simulink model "VTOL_DigitalPID"  (R2016b)
settings: Solver=ode45  StartTime=0.0  StopTime=500  RelTol=1e-3  EnableMultiTasking=on
InitFcn:
  | param
undefined symbols (not defined in the file or in its folder): drawVTOLsys, P, VTOL_ctrl_state_int
settings Model: Creator=beard  LastModifiedBy=Jacob
settings DataIOCC: LimitDataPoints=on  SaveFormat=Array  SignalLoggingSaveFormat=ModelDataLogs
settings OptimizationCC: ExpressionDepthLimit=2147483647  InitFltsAndDblsToZero=on  LifeSpan=inf
settings DebuggingCC: UnderspecifiedInitializationDetection=Classic  MergeDetectMultiDrivingBlocksExec=none  SolverPrmCheckMsg=warning  FcnCallInpInsideContextMsg=warning  StateNameClashWarn=warning  SFUnexpectedBacktrackingDiag=warning  SFNoUnconditionalDefaultTransitionDiag=warning  SFExecutionAtInitializationDiag=none
settings HardwareCC: ProdBitPerPointer=32  ProdBitPerSizeT=32  ProdBitPerPtrDiffT=32  ProdLargestAtomicFloat=None  ProdIntDivRoundTo=Undefined  ProdEndianess=Unspecified  ProdWordSize=32  ProdHWDeviceType=32-bit Generic
settings ModelReferenceCC: PropagateSignalLabelsOutOfModel=off
settings GRTTargetCC: TargetLangStandard=C89/C90 (ANSI)  GeneratePreprocessorConditionals=Disable all  CombineOutputUpdateFcns=off  GRTInterface=on
settings ConfigComp: CovMetricSettings=dw  CovHtmlReporting=on  CovSaveCumulativeToWorkspaceVar=on  CovSaveSingleToWorkspaceVar=on  CovExternalEMLEnable=off

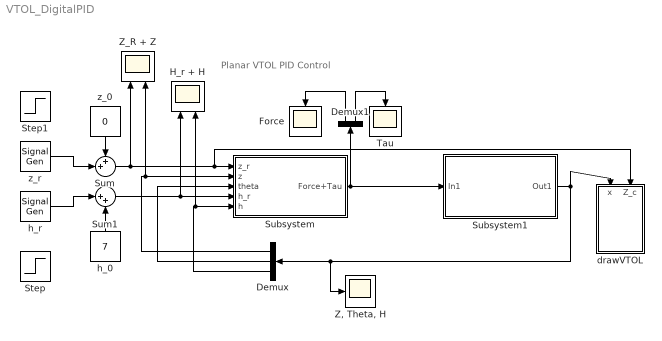
== system VTOL_DigitalPID ==
  note: Planar VTOL PID Control
  Demux : Demux  Outputs=3
  Demux1 : Demux  Outputs=2
  Force : Scope
  H_r + H : Scope  NumInputPorts=2
  Step : Step  After=3  SampleTime=0
  Step1 : Step  After=2  SampleTime=0
  Subsystem : Subsystem
  Subsystem1 : Subsystem
  Sum : Sum  Inputs=++|
  Sum1 : Sum  Inputs=|++
  Tau : Scope
  "Z, Theta, H" : Scope
  Z_R + Z : Scope  NumInputPorts=2
  drawVTOL : Subsystem
  h_0 : Constant  Value=7
  h_r : SignalGenerator  WaveForm=square  Amplitude=5  Frequency=.01
  z_0 : Constant  Value=0
  z_r : SignalGenerator  WaveForm=square  Amplitude=5  Frequency=0.015
  wires:
  z_0/1 -> Sum/1
  h_0/1 -> Sum1/2
  Sum/1 -> drawVTOL/2(Z_c), Subsystem/1(z_r), Z_R + Z/1
  Demux/1 -> Subsystem/2(z), Z_R + Z/2
  Demux/2 -> Subsystem/3(theta)
  Demux/3 -> Subsystem/5(h), H_r + H/2
  Sum1/1 -> Subsystem/4(h_r), H_r + H/1
  h_r/1 -> Sum1/1
  z_r/1 -> Sum/2
  Demux1/2 -> Tau/1
  Demux1/1 -> Force/1
  Subsystem/1(Force+Tau) -> Subsystem1/1(In1), Demux1/1
  Subsystem1/1(Out1) -> "Z, Theta, H"/1, Demux/1, drawVTOL/1(x)

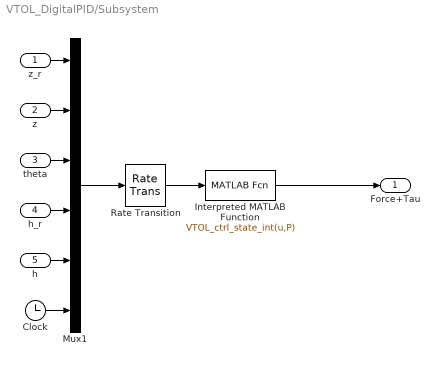
== system VTOL_DigitalPID/Subsystem ==
  z_r : Inport
  z : Inport  Port=2
  theta : Inport  Port=3
  h_r : Inport  Port=4
  h : Inport  Port=5
  Clock : Clock
  Interpreted MATLAB Function : MATLABFcn  MATLABFcn=VTOL_ctrl_state_int(u,P)  OutputDimensions=2  Output1D=off
  Mux1 : Mux  Inputs=6
  Rate Transition : RateTransition  OutPortSampleTime=P.Ts
  Force+Tau : Outport
  wires:
  Rate Transition/1 -> Interpreted MATLAB Function/1
  Mux1/1 -> Rate Transition/1
  z_r/1 -> Mux1/1
  h_r/1 -> Mux1/4
  theta/1 -> Mux1/3
  z/1 -> Mux1/2
  h/1 -> Mux1/5
  Clock/1 -> Mux1/6
  Interpreted MATLAB Function/1 -> Force+Tau/1

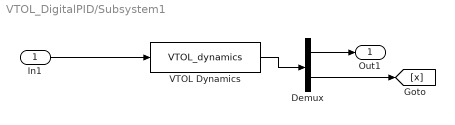
== system VTOL_DigitalPID/Subsystem1 ==
  In1 : Inport
  Demux : Demux  Outputs=2
  VTOL Dynamics : S-Function  FunctionName=VTOL_dynamics  Parameters=P  SFunctionDeploymentMode=off  EnableBusSupport=off
  Out1 : Outport
  wires:
  In1/1 -> VTOL Dynamics/1
  VTOL Dynamics/1 -> Demux/1
  Demux/1 -> Out1/1
  Demux/2 -> [x]

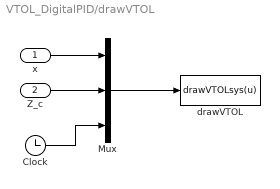
== system VTOL_DigitalPID/drawVTOL ==
  x : Inport
  Z_c : Inport  Port=2
  Clock : Clock
  Mux : Mux  Inputs=3
  drawVTOL : MATLABFcn  MATLABFcn=drawVTOLsys(u)  OutputDimensions=0  SampleTime=.5
  wires:
  Mux/1 -> drawVTOL/1
  x/1 -> Mux/1
  Clock/1 -> Mux/3
  Z_c/1 -> Mux/2
